simulink model "Task_4"  (R2016a)
settings: Solver=VariableStepAuto  StartTime=0.0  StopTime=100.0  RelTol=1e-3
undefined symbols (not defined in the file): b, J, ke, kt, L, R
libraries: simulink x1
settings Model: DataDictionary=data.sldd  Creator=Admin  LastModifiedBy=Admin

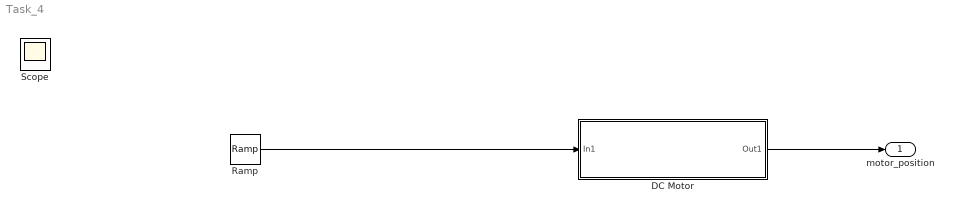
== system Task_4 ==
  "DC Motor " : Subsystem
  Ramp : simulink/Sources/Ramp  slope=1  start=0  X0=0
  motor_position : Outport
  Scope : Scope
  wires:
  "DC Motor "/1(Out1) -> motor_position/1
  Ramp/1 -> "DC Motor "/1(In1)

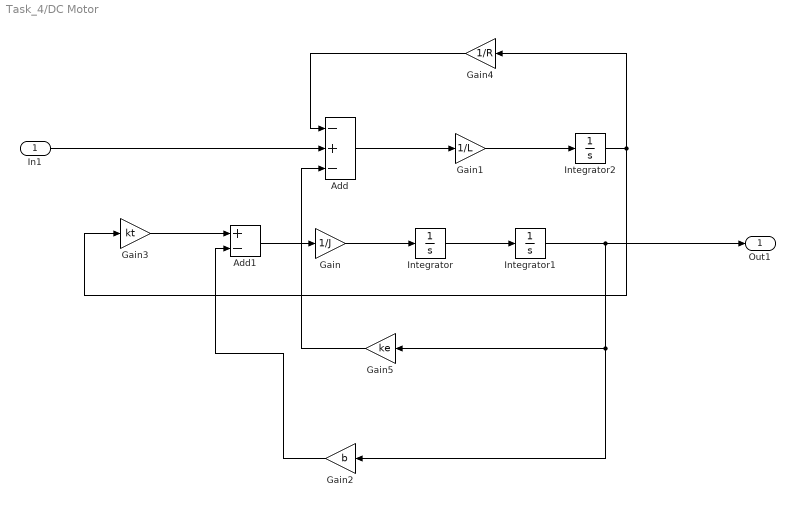
== system Task_4/DC Motor  ==
  In1 : Inport
  Add : Sum  Inputs=-+-
  Add1 : Sum  Inputs=+-
  Gain : Gain  Gain=1/J
  Gain1 : Gain  Gain=1/L
  Gain2 : Gain  Gain=b
  Gain3 : Gain  Gain=kt
  Gain4 : Gain  Gain=1/R
  Gain5 : Gain  Gain=ke
  Integrator : Integrator
  Integrator1 : Integrator
  Integrator2 : Integrator
  Out1 : Outport
  wires:
  Integrator1/1 -> Out1/1, Gain5/1, Gain2/1
  Gain/1 -> Integrator/1
  Gain3/1 -> Add1/1
  Gain1/1 -> Integrator2/1
  Add1/1 -> Gain/1
  In1/1 -> Add/2
  Integrator2/1 -> Gain3/1, Gain4/1
  Gain2/1 -> Add1/2
  Gain4/1 -> Add/1
  Integrator/1 -> Integrator1/1
  Add/1 -> Gain1/1
  Gain5/1 -> Add/3
